simulink model "WT"  (R2025a)
settings: Solver=VariableStepAuto  StartTime=0.0  StopTime=259200  FixedStep=1  MaxStep=6912.0  RelTol=1e-3  AbsTol=1e-6
model workspace (MATLAB code in the model file):
  | % load initial conditions and physical properties from file
  | 
  | sldemo_househeat_data
libraries: spsWindTurbineLib x1
Description:
  | DT model for a residential scale Wind Turbine.
  | 
  | FMI.V2 tool has been utilized for cross-platform model exchange interoperability.
  | 
  | The simulation is offline and conducted for three days.
settings Model: ExtModeTrigDuration=100  Creator=The MathWorks, Inc.  LastModifiedBy=DR53SF
settings SolverCC: AutoScaleAbsTol=off  AlgebraicLoopSolver=TrustRegion
settings DataIOCC: ExternalInput=[]  InitialState=[]
settings OptimizationCC: BlockReduction=off  BooleanDataType=off  ReuseModelBlockBuffer=off  ExpressionDepthLimit=2147483647.0  InitFltsAndDblsToZero=on  LifeSpan=inf  BufferReusableBoundary=off
settings DebuggingCC: SaveWithParameterizedLinksMsg=none  UnderspecifiedInitializationDetection=Classic  MergeDetectMultiDrivingBlocksExec=none  SignalResolutionControl=TryResolveAllWithWarning  MultiTaskDSMMsg=warning  MultiTaskCondExecSysMsg=none  IntegerOverflowMsg=none  FcnCallInpInsideContextMsg=warning  UnconnectedInputMsg=warning  UnconnectedOutputMsg=warning  UnconnectedLineMsg=warning  BusObjectLabelMismatch=none  StateNameClashWarn=warning  SFUnexpectedBacktrackingDiag=warning  SFNoUnconditionalDefaultTransitionDiag=warning  SFExecutionAtInitializationDiag=none  IntegerSaturationMsg=none  ArithmeticOperatorsInVariantConditions=warning
settings HardwareCC: ProdBitPerPointer=32.0  ProdBitPerSizeT=32.0  ProdBitPerPtrDiffT=32.0  ProdLargestAtomicFloat=None  ProdIntDivRoundTo=Undefined  ProdEndianess=Unspecified  ProdWordSize=32.0  ProdHWDeviceType=32-bit Generic  TargetUnknown=on
settings ModelReferenceCC: EnableRefExpFcnMdlSchedulingChecks=on  PropagateSignalLabelsOutOfModel=off
settings SFSimCC: SimUseLocalCustomCode=off  CustomCodeUndefinedFunction=UseInterfaceOnly
settings RTWCC: RTWUseLocalCustomCode=off  GPUComputeCapability=3.5
settings CodeAppCC: StateflowObjectComments=on
settings GRTTargetCC: TargetFcnLib=ansi_tfl_tmw.mat  TargetLangStandard=C89/C90 (ANSI)  CombineOutputUpdateFcns=off  GRTInterface=on
settings ConfigComp: CovMetricSettings=dw  CovSaveCumulativeToWorkspaceVar=on  CovSaveSingleToWorkspaceVar=on  CovExternalEMLEnable=off

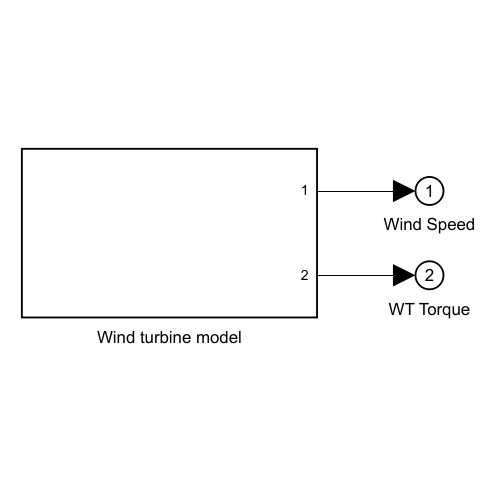
[thumbnail: Simulink's stored preview of the top-level diagram]
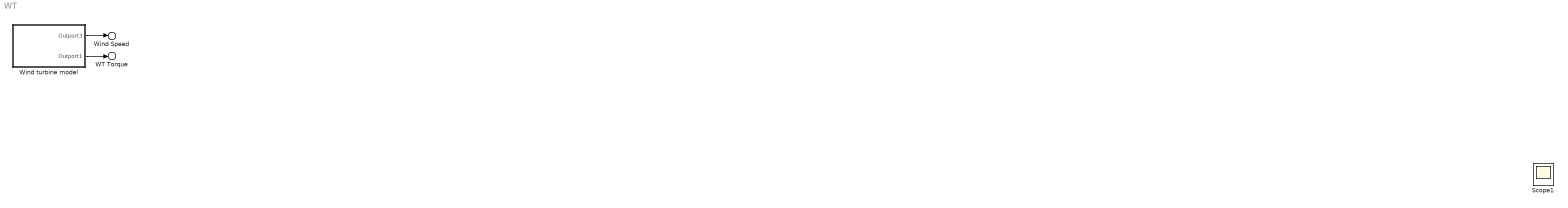
== system WT ==
  Wind turbine model : Subsystem
  Wind Speed : Outport
  WT Torque : Outport  Port=2
  Scope1 : Scope
      settings: ActiveDisplayYMinimum=-0.125  ActiveDisplayYMaximum=1.125
  wires:
  Wind turbine model/1(Outport3) -> Wind Speed/1
  Wind turbine model/2(Outport1) -> WT Torque/1

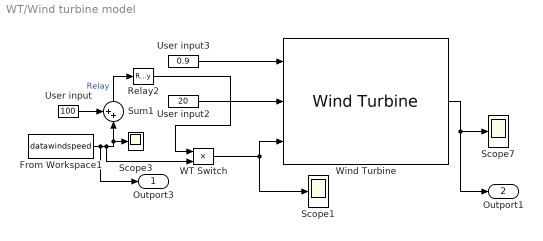
== system WT/Wind turbine model ==
  From Workspace1 : FromWorkspace  VariableName=datawindspeed
  Relay2 : Relay  OnSwitchValue=104.5  OffSwitchValue=104
  Scope1 : Scope
      settings: ActiveDisplayYMinimum=-0.91521989589008257  ActiveDisplayYMaximum=8.2369790630107449
  Scope3 : Scope
      settings: ActiveDisplayYMinimum=-0.91521989589008257  ActiveDisplayYMaximum=8.2369790630107449
  Scope7 : Scope
      settings: ActiveDisplayYMinimum=-0.0083638500969121111  ActiveDisplayYMaximum=0.00092931667743467879  DataLoggingVariableName=ScopeData3
  Sum1 : Sum  Inputs=++|  InputSameDT=on  SaturateOnIntegerOverflow=on  OutDataTypeStr=Inherit: Same as first input
  User input : Constant  Value=100
  User input2 : Constant  Value=20
  User input3 : Constant  Value=0.9
  WT Switch : Product  RndMeth=Zero
  Wind Turbine : spsWindTurbineLib/Wind Turbine  Pnom=5e3  Pelec_base=1.5e06/0.9  wind_base=2  P_wind_base=0.73  speed_nom=1.2  pitch_angle=20  c1_c6="[0.51763          116          0.4            5           21     0.006795]"  cp_nom=0.48  lambda_nom=8.1
  Outport3 : Outport
  Outport1 : Outport  Port=2
  wires:
  User input3/1 -> Wind Turbine/1
  Wind Turbine/1 -> Scope7/1, Outport1/1
  Sum1/1 -> Relay2/1  "Relay"
  From Workspace1/1 -> Outport3/1, WT Switch/2, Sum1/2, Scope3/1
  User input2/1 -> Wind Turbine/2
  User input/1 -> Sum1/1
  WT Switch/1 -> Scope1/1, Wind Turbine/3
  Relay2/1 -> WT Switch/1
